simulink model "lmsxyplot"  (Simulink 8.3)
settings: Solver=FixedStepDiscrete  StartTime=0.0  StopTime=1500  RelTol=1e-3
InitFcn:
  | w=[0.5 0.5 ones(1,18)];
  | z=zeros(1,18);
undefined symbols (not defined in the file or in its folder): dfilt, lmsxy
libraries: dspadpt3 x4, dspsrcs4 x2, dsparch4 x1, dspmisc x1
CloseFcn:
  | clear tout;
  | clear w;
  | clear z;
settings Model: Creator=The MathWorks Inc.  ExtModeAutoUpdateStatusClock=off
settings DataIOCC: SignalLoggingName=sigsOut
settings OptimizationCC: ExpressionDepthLimit=2147483647  InitFltsAndDblsToZero=on
settings DebuggingCC: SaveWithParameterizedLinksMsg=none  CheckExecutionContextPreStartOutputMsg=on  CheckExecutionContextRuntimeOutputMsg=on  SignalResolutionControl=TryResolveAllWithWarning  SolverPrmCheckMsg=none  MultiTaskDSMMsg=warning  MultiTaskCondExecSysMsg=none  FcnCallInpInsideContextMsg=UseLocalSettings  StrictBusMsg=None
settings HardwareCC: TargetUnknown=on
settings ModelReferenceCC: UpdateModelReferenceTargets=IfOutOfDate
settings RTWCC: IncludeERTFirstTime=on
settings GRTTargetCC: TargetFcnLib=ansi_tfl_tmw.mat

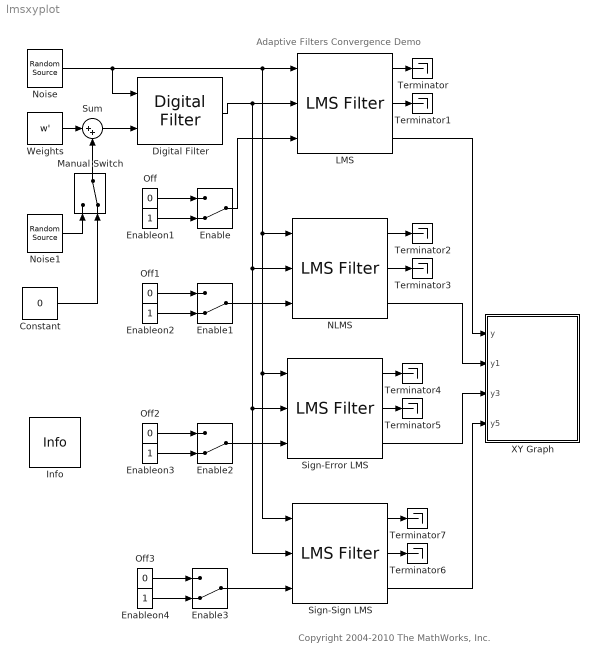
== system lmsxyplot ==
  note: Adaptive Filters Convergence Demo
  note: Copyright 2004-2010 The MathWorks, Inc.
  Constant : Constant  Value=0  VectorParams1D=off  SampleTime=1
  Digital Filter : dsparch4/Digital Filter  TypePopup=FIR (all zeros)  IIRFiltStruct=Direct form II transposed  AllPoleFiltStruct=Direct form  FIRFiltStruct=Direct form  CoeffSource=Input port(s)  NumCoeffs=[1 2]  DenCoeffs=[1 0.1]  BiQuadCoeffs=[1 0.3 0.4 1 0.1 0.2]  LatticeCoeffs=[0.2 0.4]  denIgnore=on  FiltPerSampPopup=One filter per frame  IC=0  ICnum=0  ICden=0  roundingMode=Floor  overflowMode=off  ScaleValues=0  scaleValueFracLength=14  stageInFracLength=15  stageOutFracLength=15  FilterSource=Input port(s)  dfiltObjectName=dfilt.dffir([1 2 1])
  Enable{,1..3} (4 alike) : ManualSwitch  CurrentSetting=0
  Enableon{1..4} (4 alike) : Constant  OutDataTypeStr=boolean
  Info : dspmisc/Info  SystemSampleTime=-1
  LMS : dspadpt3/LMS Filter  Algo=LMS  L=20  stepflag=Dialog  mu=0.005  leakage=1.0  ic=[0 0 z]  Adapt=on  resetflag=None  weights=on  firstCoeffMode=User-defined  firstCoeffWordLength=16  firstCoeffFracLength=15  secondCoeffMode=User-defined  secondCoeffWordLength=2  secondCoeffFracLength=15  accumMode=User-defined  accumWordLength=32  accumFracLength=20  accum2Mode=User-defined  accum2FracLength=20  prodOutputMode=User-defined  prodOutputWordLength=32  prodOutputFracLength=20  prodOutput2Mode=User-defined  prodOutput2FracLength=20  prodOutput3Mode=User-defined  prodOutput3FracLength=20  prodOutput4Mode=User-defined  prodOutput4FracLength=20  quotientMode=User-defined  quotientFracLength=20  memoryMode=User-defined  memoryWordLength=16  memoryFracLength=15  roundingMode=Nearest  overflowMode=on  addnparflag=off
  Manual Switch : ManualSwitch  CurrentSetting=0
  NLMS : dspadpt3/LMS Filter  Algo=Normalized LMS  L=20  stepflag=Dialog  mu=0.05  leakage=1.0  ic=[1 0 z]  Adapt=on  resetflag=None  weights=on  firstCoeffMode=User-defined  firstCoeffWordLength=16  firstCoeffFracLength=15  secondCoeffMode=User-defined  secondCoeffWordLength=2  secondCoeffFracLength=15  accumMode=User-defined  accumWordLength=32  accumFracLength=20  accum2Mode=User-defined  accum2FracLength=20  prodOutputMode=User-defined  prodOutputWordLength=32  prodOutputFracLength=20  prodOutput2Mode=User-defined  prodOutput2FracLength=20  prodOutput3Mode=User-defined  prodOutput3FracLength=20  prodOutput4Mode=User-defined  prodOutput4FracLength=20  quotientMode=User-defined  quotientFracLength=20  memoryMode=User-defined  memoryWordLength=16  memoryFracLength=15  roundingMode=Nearest  overflowMode=on  addnparflag=off
  Noise : dspsrcs4/Random Source  SrcType=Gaussian  NormMethod=Ziggurat  CltLength=12  MinVal=0  MaxVal=1  MeanVal=0  VarVal=1  RepMode=Specify seed  rawSeed=[23341]  IsInherit=off  SampMode=Discrete  SampTime=1  SampFrame=1  DataType=Double  OutComplex=Real
  Noise1 : dspsrcs4/Random Source  SrcType=Gaussian  NormMethod=Ziggurat  CltLength=12  MinVal=0  MaxVal=1  MeanVal=0  VarVal=0.01  RepMode=Specify seed  rawSeed=[23341]  IsInherit=off  SampMode=Discrete  SampTime=1/20  SampFrame=20  DataType=Double  OutComplex=Real
  Off{,1..3} (4 alike) : Constant  Value=0  OutDataTypeStr=boolean
  Sign-Error LMS : dspadpt3/LMS Filter  Algo=Sign-Error LMS  L=20  stepflag=Dialog  mu=0.005  leakage=1.0  ic=[0 1 z]  Adapt=on  resetflag=None  weights=on  firstCoeffMode=User-defined  firstCoeffWordLength=16  firstCoeffFracLength=15  secondCoeffMode=User-defined  secondCoeffWordLength=2  secondCoeffFracLength=15  accumMode=User-defined  accumWordLength=32  accumFracLength=20  accum2Mode=User-defined  accum2FracLength=20  prodOutputMode=User-defined  prodOutputWordLength=32  prodOutputFracLength=20  prodOutput2Mode=User-defined  prodOutput2FracLength=20  prodOutput3Mode=User-defined  prodOutput3FracLength=20  prodOutput4Mode=User-defined  prodOutput4FracLength=20  quotientMode=User-defined  quotientFracLength=20  memoryMode=User-defined  memoryWordLength=16  memoryFracLength=15  roundingMode=Nearest  overflowMode=on  addnparflag=off
  Sign-Sign LMS : dspadpt3/LMS Filter  Algo=Sign-Sign LMS  L=20  stepflag=Dialog  mu=0.005  leakage=1.0  ic=[1 1 z]  Adapt=on  resetflag=None  weights=on  firstCoeffMode=User-defined  firstCoeffWordLength=16  firstCoeffFracLength=15  secondCoeffMode=User-defined  secondCoeffWordLength=2  secondCoeffFracLength=15  accumMode=User-defined  accumWordLength=32  accumFracLength=20  accum2Mode=User-defined  accum2FracLength=20  prodOutputMode=User-defined  prodOutputWordLength=32  prodOutputFracLength=20  prodOutput2Mode=User-defined  prodOutput2FracLength=20  prodOutput3Mode=User-defined  prodOutput3FracLength=20  prodOutput4Mode=User-defined  prodOutput4FracLength=20  quotientMode=User-defined  quotientFracLength=20  memoryMode=User-defined  memoryWordLength=16  memoryFracLength=15  roundingMode=Nearest  overflowMode=on  addnparflag=off
  Sum : Sum  Inputs=|++  SaturateOnIntegerOverflow=on
  Terminator{,1..7} (8 alike) : Terminator
  Weights : Constant  Value=w'  VectorParams1D=off  SampleTime=1
  XY Graph : Subsystem  LoadFcn=lmsxy([],[],[],'LoadBlock',[])  StopFcn=lmsxy([],[],[],'Stop',[])  TreatAsAtomicUnit=on  SimViewingDevice=on  mask(XY-Scope){xmin=0, xmax=1, ymin=0, ymax=1, st=-1, R=[0 1], W=w}
      mask prompts: xmin "x-min:"; xmax "x-max:"; ymin "y-min:"; ymax "y-max:"; st "Sample time:"; R "Input parameters [mean variance]"; W "Weights"
      mask help: XY scope using MATLAB graph window. First input is used as time base. Enter plotting ranges.
      mask init:
      | lmsxy([],[],[],'Start', [R W(1:2) xmin xmax ymin ymax])
      settings: CopyFcn=lmsxy([],[],[],'CopyBlock',[])  DeleteFcn=lmsxy([],[],[],'DeleteBlock',[])  NameChangeFcn=lmsxy([],[],[],'NameChange',[])
      mask Help: This block can be used to explore limit cycles. Look at the MATLAB file sfunxy.m to see how it works.
      mask Display: plot([.05 .95 .95 .05 .05],[.45 .45 .95 .95 .45], 0.5+cos(0:0.1:2*pi)*0.3,0.7+sin(0:0.1:2*pi)*0.2)
  wires:
  Noise/1 -> LMS/1, NLMS/1, Sign-Error LMS/1, Sign-Sign LMS/1, Digital Filter/1
  Digital Filter/1 -> LMS/2, NLMS/2, Sign-Error LMS/2, Sign-Sign LMS/2
  LMS/1 -> Terminator/1
  LMS/2 -> Terminator1/1
  LMS/3 -> XY Graph/1(y)
  NLMS/3 -> XY Graph/2(y1)
  Sign-Error LMS/3 -> XY Graph/3(y3)
  NLMS/1 -> Terminator2/1
  NLMS/2 -> Terminator3/1
  Sign-Error LMS/1 -> Terminator4/1
  Sign-Error LMS/2 -> Terminator5/1
  Sign-Sign LMS/2 -> Terminator6/1
  Sign-Sign LMS/1 -> Terminator7/1
  Enable/1 -> LMS/3
  Enable1/1 -> NLMS/3
  Enable3/1 -> Sign-Sign LMS/3
  Sum/1 -> Digital Filter/2
  Weights/1 -> Sum/1
  Manual Switch/1 -> Sum/2
  Noise1/1 -> Manual Switch/1
  Constant/1 -> Manual Switch/2
  Off/1 -> Enable/1
  Enableon1/1 -> Enable/2
  Off1/1 -> Enable1/1
  Enableon2/1 -> Enable1/2
  Enable2/1 -> Sign-Error LMS/3
  Off2/1 -> Enable2/1
  Enableon3/1 -> Enable2/2
  Off3/1 -> Enable3/1
  Enableon4/1 -> Enable3/2
  Sign-Sign LMS/3 -> XY Graph/4(y5)

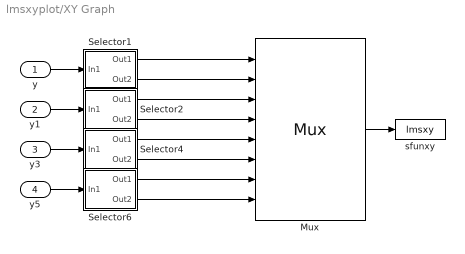
== system lmsxyplot/XY Graph ==
  y : Inport
  y1 : Inport  Port=2
  y3 : Inport  Port=3
  y5 : Inport  Port=4
  Mux : Mux  Inputs=8
  Selector1 : Subsystem
  Selector2 : Subsystem
  Selector4 : Subsystem
  Selector6 : Subsystem
  sfunxy : S-Function  FunctionName=lmsxy  Parameters=[xmin xmax ymin ymax 1:6], st  EnableBusSupport=off
  wires:
  Selector1/2(Out2) -> Mux/2
  Mux/1 -> sfunxy/1
  Selector1/1(Out1) -> Mux/1
  Selector2/1(Out1) -> Mux/3
  Selector2/2(Out2) -> Mux/4
  Selector4/1(Out1) -> Mux/5
  Selector4/2(Out2) -> Mux/6
  Selector6/1(Out1) -> Mux/7
  Selector6/2(Out2) -> Mux/8
  y/1 -> Selector1/1(In1)
  y1/1 -> Selector2/1(In1)
  y3/1 -> Selector4/1(In1)
  y5/1 -> Selector6/1(In1)

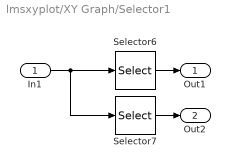
== system lmsxyplot/XY Graph/Selector1 ==
  In1 : Inport
  Selector6 : Selector  Indices=2
  Selector7 : Selector
  Out1 : Outport
  Out2 : Outport  Port=2
  wires:
  Selector7/1 -> Out2/1
  Selector6/1 -> Out1/1
  In1/1 -> Selector7/1, Selector6/1

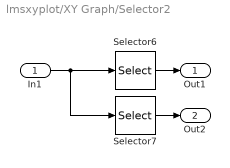
== system lmsxyplot/XY Graph/Selector2 ==
  In1 : Inport
  Selector6 : Selector  Indices=2
  Selector7 : Selector
  Out1 : Outport
  Out2 : Outport  Port=2
  wires:
  Selector7/1 -> Out2/1
  Selector6/1 -> Out1/1
  In1/1 -> Selector7/1, Selector6/1

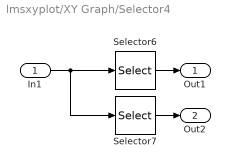
== system lmsxyplot/XY Graph/Selector4 ==
  In1 : Inport
  Selector6 : Selector  Indices=2
  Selector7 : Selector
  Out1 : Outport
  Out2 : Outport  Port=2
  wires:
  In1/1 -> Selector6/1, Selector7/1
  Selector6/1 -> Out1/1
  Selector7/1 -> Out2/1

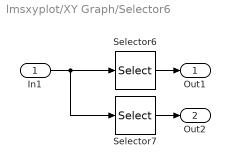
== system lmsxyplot/XY Graph/Selector6 ==
  In1 : Inport
  Selector6 : Selector  Indices=2
  Selector7 : Selector
  Out1 : Outport
  Out2 : Outport  Port=2
  wires:
  Selector7/1 -> Out2/1
  Selector6/1 -> Out1/1
  In1/1 -> Selector7/1, Selector6/1
